simulink model "mophongstimulink"  (R2025a)
settings: Solver=FixedStepAuto  StartTime=0.0  StopTime=60  FixedStep=0.01  RelTol=1e-3
values from neighbouring files (symbols this model uses):
  A = zeros(4,4)    [mophongmatlab.m]
  B = zeros(4,1)    [mophongmatlab.m]
  C = eye(4)    [mophongmatlab.m]
  D = zeros(4,1)    [mophongmatlab.m]
undefined symbols (not defined in the file or in its folder): K_opt
settings Model: Creator=ADMIN  LastModifiedBy=ADMIN

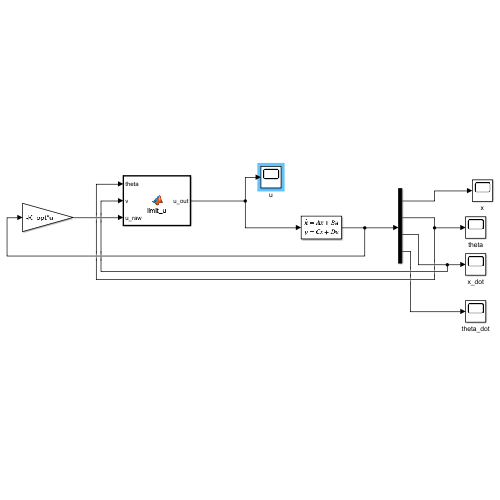
[thumbnail: Simulink's stored preview of the top-level diagram]
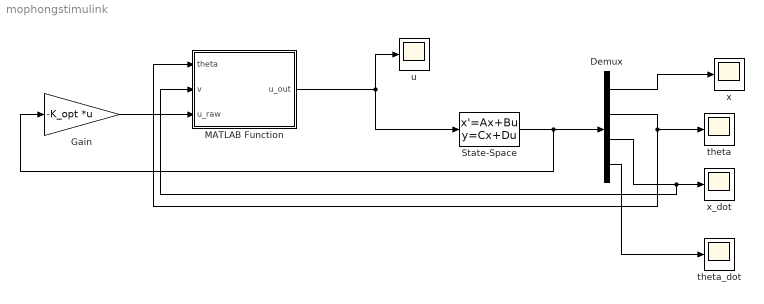
== system mophongstimulink ==
  Demux : Demux
  Gain : Gain  Gain=-K_opt  Multiplication=Matrix(K*u)
  MATLAB Function : MATLAB Function  TreatAsAtomicUnit=on
  State-Space : StateSpace  A=A  B=B  C=C  D=D  InitialCondition=[0,15*pi/180,0,0]
  theta : Scope
      settings: ActiveDisplayYMinimum=-0.2077395510704515  ActiveDisplayYMaximum=0.28051949037404639
  theta_dot : Scope
      settings: ActiveDisplayYMinimum=-0.88353532650428956  ActiveDisplayYMaximum=0.19427003367989115  DataLoggingVariableName=ScopeData3
  u : Scope
      settings: ActiveDisplayYMinimum=-2.6609648422539895  ActiveDisplayYMaximum=2.5251727458291651  DataLoggingVariableName=ScopeData4
  x : Scope
      settings: ActiveDisplayYMinimum=-0.03695393895183971  ActiveDisplayYMaximum=0.26188493078308928
  x_dot : Scope
      settings: ActiveDisplayYMinimum=-0.11154537524990757  ActiveDisplayYMaximum=0.25451100662754389  DataLoggingVariableName=ScopeData2
  wires:
  State-Space/1 -> Demux/1, Gain/1
  MATLAB Function/1(u_out) -> State-Space/1, u/1
  Gain/1 -> MATLAB Function/3(u_raw)
  Demux/1 -> x/1
  Demux/2 -> MATLAB Function/1(theta), theta/1
  Demux/3 -> MATLAB Function/2(v), x_dot/1
  Demux/4 -> theta_dot/1

== matlab function mophongstimulink/MATLAB Function ==
  data: theta input; v input; u_out output; u_raw input
function u_out = limit_u(theta, v, u_raw)

% Gioi han
u_max = 12;      % N.m
v_max = 0.6;     % m/s
a_max = 2.0;     % m/s^2, dung cho goc ban dau 15 do

% Gia tri lay tu ma tran A, B cua mo hinh
A32 = -5.71394429;
B3  = -1.74651380;

% Gia toc tu nhien do goc nghieng
a_free = A32 * theta;

% Gioi han gia toc
a_low  = -a_max;
a_high =  a_max;

% Neu van toc da cham gioi han thi khong cho tang toc tiep
if v >= v_max
    a_high = min(a_high, 0);
elseif v <= -v_max
    a_low = max(a_low, 0);
end

% Tim khoang u sao cho:
% a_low <= A32*theta + B3*u <= a_high
u1 = (a_low  - a_free) / B3;
u2 = (a_high - a_free) / B3;

u_low  = min(u1, u2);
u_high = max(u1, u2);

% Gioi han theo gia toc
u_out = min(max(u_raw, u_low), u_high);

% Gioi han theo moment dong co
u_out = min(max(u_out, -u_max), u_max);

end
